simulink model "extractLocalMap_simfcnsvr"  (R2024b)
settings: Solver=FixedStepAuto  StartTime=0.0  StopTime=10.0  RelTol=1e-3
undefined symbols (not defined in the file): maxLocalPathLen, maxRefPathLen
libraries: simulink x2
settings Model: Creator=cstabile  LastModifiedBy=jbrault
settings SolverCC: DateTimeAtSimulationTimeZero=[]
settings SFSimCC: SimTargetLang=C++

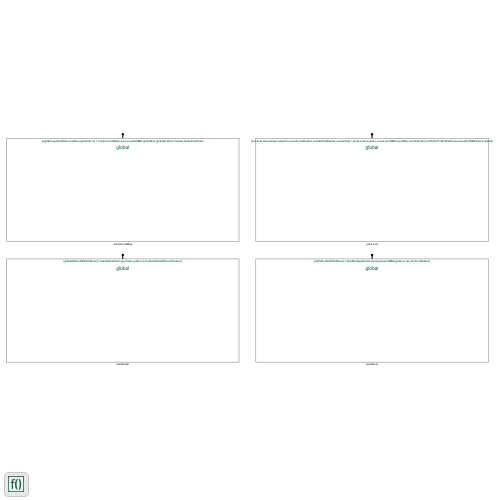
[thumbnail: Simulink's stored preview of the top-level diagram]
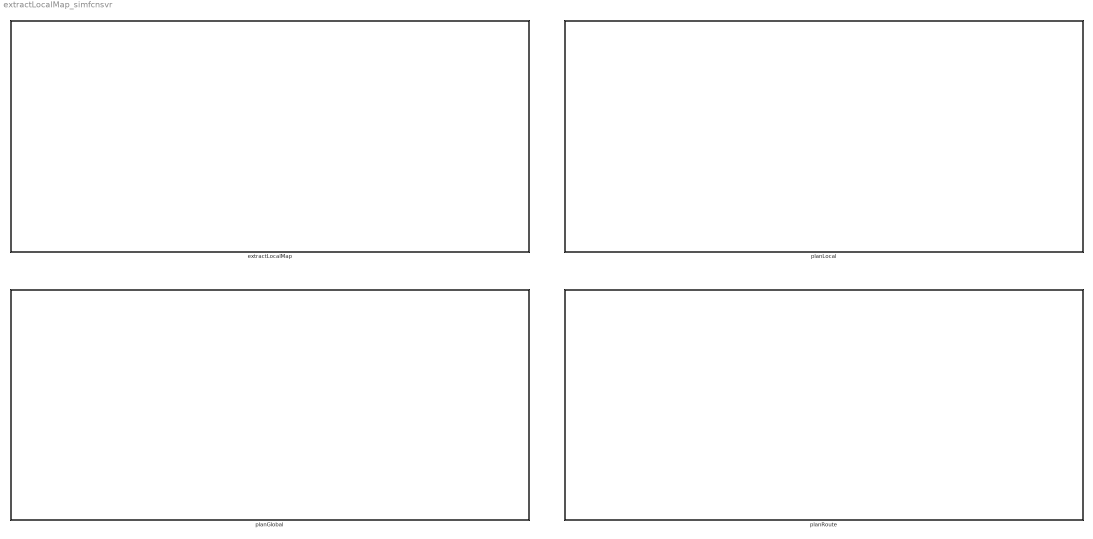
== system extractLocalMap_simfcnsvr ==
  extractLocalMap : Subsystem  TreatAsAtomicUnit=on
  planGlobal : Subsystem  TreatAsAtomicUnit=on
  planLocal : Subsystem  TreatAsAtomicUnit=on
  planRoute : Subsystem  TreatAsAtomicUnit=on

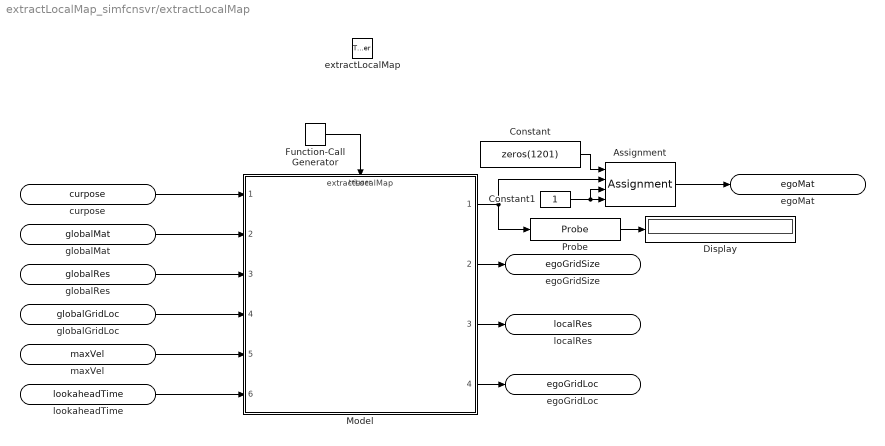
== system extractLocalMap_simfcnsvr/extractLocalMap ==
  extractLocalMap : TriggerPort  TriggerType=function-call  IsSimulinkFunction=on  FunctionName=extractLocalMap  ScopeName=global  VariantControl=(inherit)
  Assignment : Assignment  NumberOfDimensions=2  DiagnosticForDimensions=Warning  IndexOptions=Starting index (port),Starting index (port)  Indices=1,1  OutputSizes=1201,1
  Constant : Constant  Value=zeros(1201)  OutDataTypeStr=boolean
  Constant1 : Constant
  Display : Display
  Function-Call Generator : simulink/Ports & Subsystems/Function-Call Generator  sample_time=-1  numberOfIterations=1  DisallowWideOutput=off
  Model : ModelReference  ModelNameDialog=extractLocalMap.slx  SimulationMode=Normal  ModelReferenceVersion=1.0  TriggerPortName=function  TriggerPortTriggerType=function-call  TriggerPortStatesWhenEnabling=held
  Probe : Probe  ProbeWidth=off  ProbeSampleTime=off  ProbeComplexSignal=off  ProbeSignalDimensions=on
  curpose : ArgIn  DisableCoverage=on  PortDimensions=[1 3]  ArgumentName=curpose
  globalMat : ArgIn  DisableCoverage=on  Port=2  OutDataTypeStr=boolean  PortDimensions=[1201 1201]  ArgumentName=globalMat
  globalRes : ArgIn  DisableCoverage=on  Port=3  ArgumentName=globalRes
  globalGridLoc : ArgIn  DisableCoverage=on  Port=4  PortDimensions=[1 2]  ArgumentName=globalGridLoc
  maxVel : ArgIn  DisableCoverage=on  Port=5  ArgumentName=maxVel
  lookaheadTime : ArgIn  DisableCoverage=on  Port=6  ArgumentName=lookaheadTime
  egoMat : ArgOut  DisableCoverage=on  OutDataTypeStr=boolean  PortDimensions=[1201 1201]  ArgumentName=egoMat
  egoGridSize : ArgOut  DisableCoverage=on  Port=2  PortDimensions=[1 2]  ArgumentName=egoGridSize
  localRes : ArgOut  DisableCoverage=on  Port=3  ArgumentName=localRes
  egoGridLoc : ArgOut  DisableCoverage=on  Port=4  PortDimensions=[1 2]  ArgumentName=egoGridLoc
  wires:
  Model/3 -> localRes/1
  Model/2 -> egoGridSize/1
  Function-Call Generator/1 -> Model/Trigger
  curpose/1 -> Model/1
  globalGridLoc/1 -> Model/4
  lookaheadTime/1 -> Model/6
  globalRes/1 -> Model/3
  maxVel/1 -> Model/5
  globalMat/1 -> Model/2
  Model/4 -> egoGridLoc/1
  Model/1 -> Probe/1, Assignment/2
  Assignment/1 -> egoMat/1
  Constant/1 -> Assignment/1
  Constant1/1 -> Assignment/3, Assignment/4
  Probe/1 -> Display/1

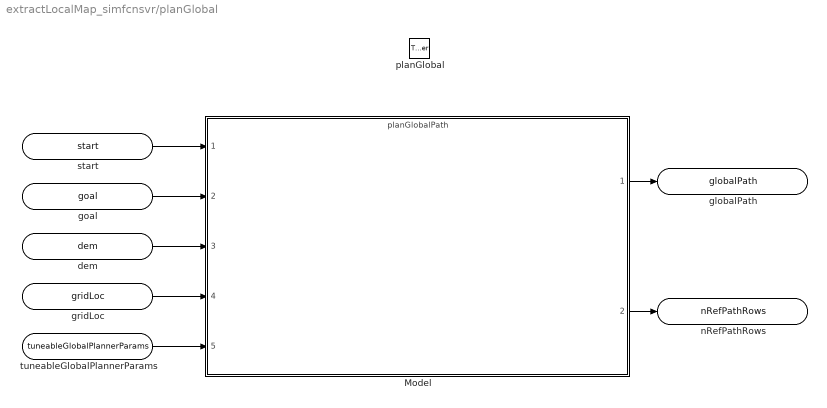
== system extractLocalMap_simfcnsvr/planGlobal ==
  planGlobal : TriggerPort  TriggerType=function-call  IsSimulinkFunction=on  FunctionName=planGlobal  VariantControl=(inherit)
  Model : ModelReference  ModelNameDialog=planGlobalPath.slx  SimulationMode=Normal  ModelReferenceVersion=1.0
  start : ArgIn  PortDimensions=[1 3]  ArgumentName=start
  goal : ArgIn  Port=2  PortDimensions=[1 3]  ArgumentName=goal
  dem : ArgIn  Port=3  OutDataTypeStr=single  PortDimensions=[1201 1201]  ArgumentName=dem
  gridLoc : ArgIn  Port=4  PortDimensions=[1 2]  ArgumentName=gridLoc
  tuneableGlobalPlannerParams : ArgIn  Port=5  OutDataTypeStr=Bus: fsp_tunable_bus  ArgumentName=tuneableGlobalPlannerParams
  globalPath : ArgOut  PortDimensions=[maxRefPathLen 3]  ArgumentName=globalPath
  nRefPathRows : ArgOut  Port=2  ArgumentName=nRefPathRows
  wires:
  Model/1 -> globalPath/1
  start/1 -> Model/1
  Model/2 -> nRefPathRows/1
  goal/1 -> Model/2
  dem/1 -> Model/3
  gridLoc/1 -> Model/4
  tuneableGlobalPlannerParams/1 -> Model/5

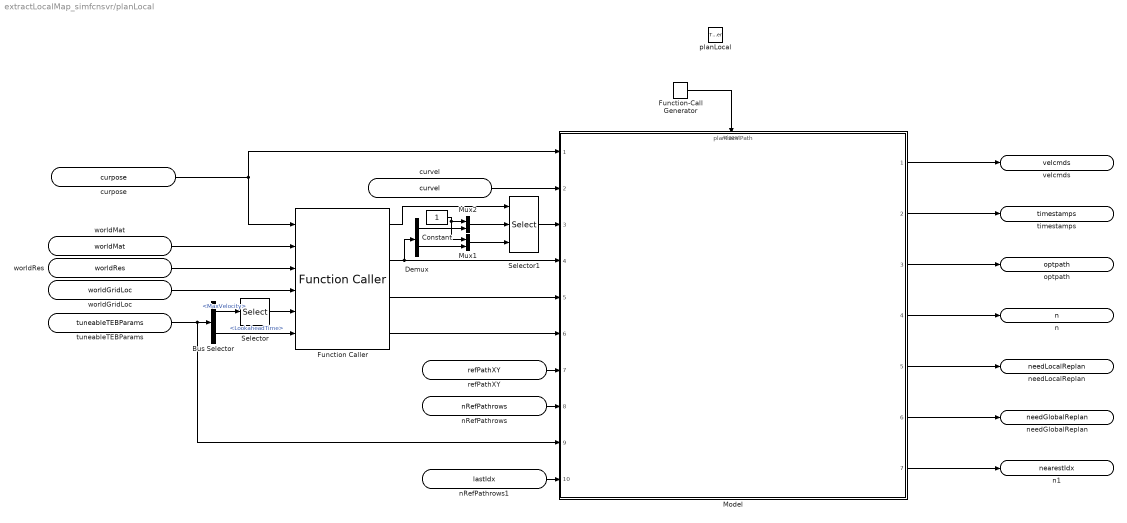
== system extractLocalMap_simfcnsvr/planLocal ==
  planLocal : TriggerPort  TriggerType=function-call  IsSimulinkFunction=on  FunctionName=planLocal  VariantControl=(inherit)
  Bus Selector : BusSelector  OutputSignals=MaxVelocity,LookaheadTime
  Constant : Constant
  Demux : Demux  Outputs=2
  Function Caller : FunctionCaller  FunctionPrototype=[egoMat,egoGridSize,localRes,egoGridLoc] = extractLocalMap(curpose,globalMat,globalRes,globalGridLoc,maxVel,lookaheadTime)  InputArgumentSpecifications=<Enter example>  OutputArgumentSpecifications=<Enter example>
  Function-Call Generator : simulink/Ports & Subsystems/Function-Call Generator  sample_time=-1  numberOfIterations=1  DisallowWideOutput=off
  Model : ModelReference  ModelNameDialog=planLocalPath.slx  SimulationMode=Normal  ModelReferenceVersion=2.0  TriggerPortName=function  TriggerPortTriggerType=function-call  TriggerPortStatesWhenEnabling=held
  Mux1 : Mux  Inputs=2
  Mux2 : Mux  Inputs=2
  Selector : Selector  InputPortWidth=2  IndexOptions=Index vector (dialog)  Indices=1  OutputSizes=1
  Selector1 : Selector  NumberOfDimensions=2  InputPortWidth=3  IndexOptions=Starting and ending indices (port),Starting and ending indices (port)  Indices=[1 3],1  OutputSizes=1,1
  curpose : ArgIn  DisableCoverage=on  PortDimensions=[1 3]  ArgumentName=curpose
  curvel : ArgIn  DisableCoverage=on  Port=2  PortDimensions=[1 2]  ArgumentName=curvel
  worldMat : ArgIn  DisableCoverage=on  Port=3  OutDataTypeStr=boolean  PortDimensions=[1201 1201]  ArgumentName=worldMat
  worldRes : ArgIn  DisableCoverage=on  Port=4  ArgumentName=worldRes
  worldGridLoc : ArgIn  DisableCoverage=on  Port=5  PortDimensions=[1 2]  ArgumentName=worldGridLoc
  refPathXY : ArgIn  DisableCoverage=on  Port=6  PortDimensions=[maxRefPathLen 3]  ArgumentName=refPathXY
  nRefPathrows : ArgIn  DisableCoverage=on  Port=7  ArgumentName=nRefPathrows
  tuneableTEBParams : ArgIn  DisableCoverage=on  Port=8  OutDataTypeStr=Bus: teb_bus  ArgumentName=tuneableTEBParams
  nRefPathrows1 : ArgIn  DisableCoverage=on  Port=9  ArgumentName=lastIdx
  velcmds : ArgOut  DisableCoverage=on  PortDimensions=[maxLocalPathLen 2]  ArgumentName=velcmds
  timestamps : ArgOut  DisableCoverage=on  Port=2  PortDimensions=[maxLocalPathLen 1]  ArgumentName=timestamps
  optpath : ArgOut  DisableCoverage=on  Port=3  PortDimensions=[maxLocalPathLen 3]  ArgumentName=optpath
  n : ArgOut  DisableCoverage=on  Port=4  ArgumentName=n
  needLocalReplan : ArgOut  DisableCoverage=on  Port=5  ArgumentName=needLocalReplan
  needGlobalReplan : ArgOut  DisableCoverage=on  Port=6  ArgumentName=needGlobalReplan
  n1 : ArgOut  DisableCoverage=on  Port=7  ArgumentName=nearestIdx
  wires:
  curpose/1 -> Model/1, Function Caller/1
  curvel/1 -> Model/2
  Model/6 -> needGlobalReplan/1
  Function Caller/2 -> Demux/1, Model/4
  nRefPathrows/1 -> Model/8
  worldMat/1 -> Function Caller/2
  refPathXY/1 -> Model/7
  worldGridLoc/1 -> Function Caller/4
  worldRes/1 -> Function Caller/3
  tuneableTEBParams/1 -> Bus Selector/1, Model/9
  Model/1 -> velcmds/1
  Model/2 -> timestamps/1
  Model/3 -> optpath/1
  Model/4 -> n/1
  Model/5 -> needLocalReplan/1
  Function-Call Generator/1 -> Model/Trigger
  Bus Selector/1 -> Selector/1  "<MaxVelocity>"
  Selector/1 -> Function Caller/5
  Bus Selector/2 -> Function Caller/6  "<LookaheadTime>"
  Function Caller/1 -> Selector1/1
  Function Caller/3 -> Model/5
  Function Caller/4 -> Model/6
  Selector1/1 -> Model/3
  Constant/1 -> Mux2/1, Mux1/1
  Demux/1 -> Mux2/2
  Mux2/1 -> Selector1/2
  Demux/2 -> Mux1/2
  Mux1/1 -> Selector1/3
  Model/7 -> n1/1
  nRefPathrows1/1 -> Model/10

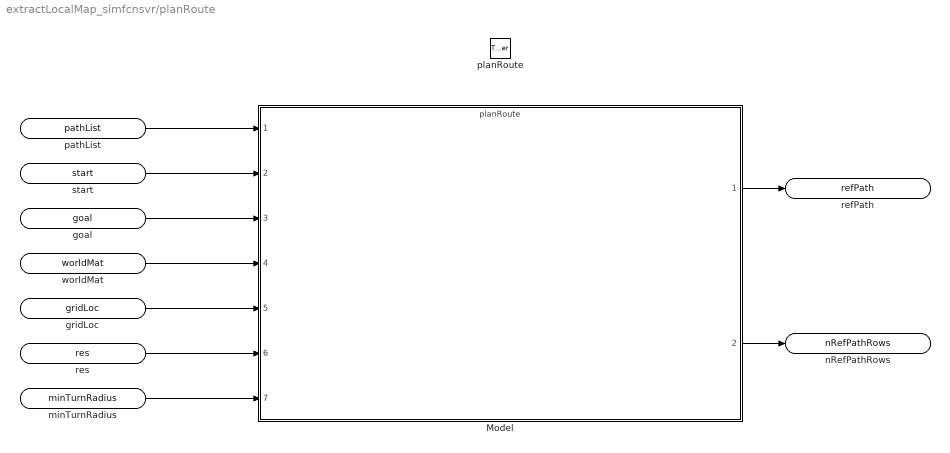
== system extractLocalMap_simfcnsvr/planRoute ==
  planRoute : TriggerPort  TriggerType=function-call  IsSimulinkFunction=on  FunctionName=planRoute  VariantControl=(inherit)
  Model : ModelReference  ModelNameDialog=planRoute.slx  SimulationMode=Normal  ModelReferenceVersion=2.0
  pathList : ArgIn  DisableCoverage=on  OutDataTypeStr=Bus: pathList_fixed_bus  ArgumentName=pathList
  start : ArgIn  DisableCoverage=on  Port=2  PortDimensions=[1 3]  ArgumentName=start
  goal : ArgIn  DisableCoverage=on  Port=3  PortDimensions=[1 3]  ArgumentName=goal
  worldMat : ArgIn  DisableCoverage=on  Port=4  OutDataTypeStr=boolean  PortDimensions=[1201 1201]  ArgumentName=worldMat
  gridLoc : ArgIn  DisableCoverage=on  Port=5  PortDimensions=[1 2]  ArgumentName=gridLoc
  res : ArgIn  DisableCoverage=on  Port=6  ArgumentName=res
  minTurnRadius : ArgIn  DisableCoverage=on  Port=7  ArgumentName=minTurnRadius
  refPath : ArgOut  DisableCoverage=on  PortDimensions=[maxRefPathLen 3]  ArgumentName=refPath
  nRefPathRows : ArgOut  DisableCoverage=on  Port=2  ArgumentName=nRefPathRows
  wires:
  pathList/1 -> Model/1
  Model/1 -> refPath/1
  Model/2 -> nRefPathRows/1
  start/1 -> Model/2
  goal/1 -> Model/3
  worldMat/1 -> Model/4
  gridLoc/1 -> Model/5
  res/1 -> Model/6
  minTurnRadius/1 -> Model/7
